simulink model "V10MODE_TEST"  (R2020b)
settings: Solver=VariableStepAuto  StartTime=0.0  StopTime=10.0  RelTol=1e-3
values from neighbouring files (symbols this model uses):
  HD = 180/pi    (= 57.2957795131)    [mode_data.m]
settings Model: Creator=a4327481  LastModifiedBy=a4327481

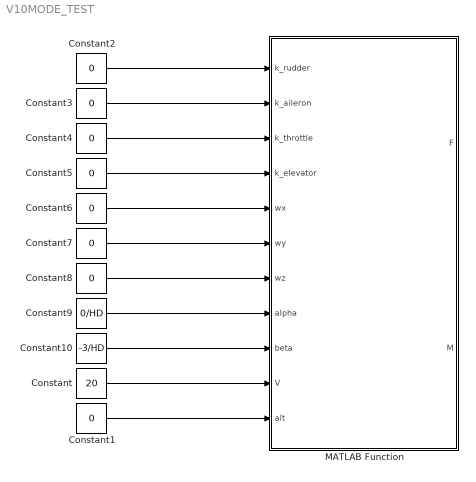
== system V10MODE_TEST ==
  Constant : Constant  Value=20
  Constant{1..8} (8 alike) : Constant  Value=0
  Constant10 : Constant  Value=-3/HD
  Constant9 : Constant  Value=0/HD
  MATLAB Function : MATLAB Function  TreatAsAtomicUnit=on
  wires:
  Constant/1 -> MATLAB Function/10(V)
  Constant1/1 -> MATLAB Function/11(alt)
  Constant2/1 -> MATLAB Function/1(k_rudder)
  Constant3/1 -> MATLAB Function/2(k_aileron)
  Constant4/1 -> MATLAB Function/3(k_throttle)
  Constant5/1 -> MATLAB Function/4(k_elevator)
  Constant6/1 -> MATLAB Function/5(wx)
  Constant7/1 -> MATLAB Function/6(wy)
  Constant8/1 -> MATLAB Function/7(wz)
  Constant10/1 -> MATLAB Function/9(beta)
  Constant9/1 -> MATLAB Function/8(alpha)

== matlab function V10MODE_TEST/MATLAB Function ==
  data: k_rudder input; k_aileron input; k_throttle input; k_elevator input; wx input; wy input; wz input; alpha input; beta input; V input; alt input; Aero parameter; F output; M output
function [F,M] = fcn(k_rudder,k_aileron,k_throttle,k_elevator,wx,wy,wz,alpha,beta,V,alt, Aero)
% 
HD=180/pi;
[~,~,rho,~] = atom_mode(alt+2000);
rho=1.225;
q=0.5*rho*V*V;
alpha=constrain_value(alpha,-10/HD,12/HD);
beta=constrain_value(beta,-10/HD,12/HD);
Sbw=[cos(alpha)*cos(beta)   -cos(alpha)*sin(beta)   -sin(alpha)
    sin(beta)               cos(beta)               0
    sin(alpha)*cos(beta)    -sin(alpha)*sin(beta)   cos(alpha)];
alpha=alpha*HD;
beta =beta* HD;
CL=interp1(Aero.CL_alpha,Aero.CL,alpha);
CD=interp1(Aero.CD_alpha,Aero.CD,alpha);
CC_beta=interp1(Aero.CC_beta,Aero.CC,abs(beta))*sign(beta);
CC=CC_beta+Aero.CC_dr*k_rudder;
D=q*Aero.Sref*CD;
C=q*Aero.Sref*CC;
L=q*Aero.Sref*CL;
Fw=[D; C; L];
Fb=Sbw*-Fw;
TF=k_throttle*Aero.Tmax;
F_Plane=Fb+[TF;0;0];
%%%%%%%%%%%%%%%%%%%%%%%%%%%%%%%%%%%%%%%%%%%%%%%%%%%%%%%%
Cm_V=interp1(Aero.Cm_alpha,Aero.Cm_V,alpha);
Cm_H=interp1(Aero.Cm_alpha,Aero.Cm_H,alpha);
Cm_L=interp1(Aero.Cm_alpha,Aero.Cm_L,alpha);
Cm_F=interp1(Aero.Cm_alpha,Aero.Cm_F,alpha);
Cm_H_de=interp1(Aero.Cm_elevator,Aero.Cm_H_de,k_elevator);
Cm=Cm_V+Cm_H+Cm_L+Cm_F+Cm_H_de;

Cl_beta=interp1(Aero.beta,Aero.Cl_beta,abs(beta))*sign(beta);
Cl_da=Aero.Cl_da*k_aileron;
Cl=Cl_beta+Cl_da;

Cn_beta=interp1(Aero.beta,Aero.Cn_beta,abs(beta))*sign(beta);
Cn_dr=Aero.Cn_dr*k_rudder;
Cn=Cn_beta+Cn_dr;

l=q*Aero.Sref*Aero.Lref*Cl-0.1*wx;
m=q*Aero.Sref*Aero.Lref*Cm-0.2*wy;
n=q*Aero.Sref*Aero.Lref*Cn-0.2*wz;
M_Plane=[l m n];

F=F_Plane;
M=M_Plane;

end
